simulink model "Logic122"  (R2016b)
settings: Solver=VariableStepAuto  StartTime=0.0  StopTime=10.0  RelTol=1e-3
settings Model: Creator=viett  LastModifiedBy=viett

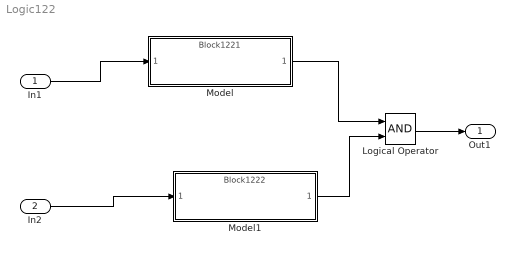
== system Logic122 ==
  In1 : Inport
  In2 : Inport  Port=2
  Logical Operator : Logic  AllPortsSameDT=off  OutDataTypeStr=boolean
  Model : ModelReference  ModelNameDialog=Block1221.slx  SimulationMode=Normal  ModelReferenceVersion=1.1
  Model1 : ModelReference  ModelNameDialog=Block1222.slx  SimulationMode=Normal  ModelReferenceVersion=1.1
  Out1 : Outport
  wires:
  Model/1 -> Logical Operator/1
  Model1/1 -> Logical Operator/2
  Logical Operator/1 -> Out1/1
  In1/1 -> Model/1
  In2/1 -> Model1/1
